simulink model "statsdem"  (Simulink 4.00)
settings: Solver=FixedStepDiscrete  StartTime=0.0  StopTime=inf  RelTol=1e-3  AbsTol=1e-6
libraries: dspbuff3 x4, dspstat3 x3, dspsrcs3 x2
settings Model: Creator=don  LastModifiedBy=schim  SaveTime=off  SaveOutput=off  LimitDataPoints=off  IntegerOverflowMsg=none  RTWOptions=-aRollThreshold=2  ExtModeTrigMode=oneshot  ExtModeArmWhenConnect=off  BlockReductionOpt=off

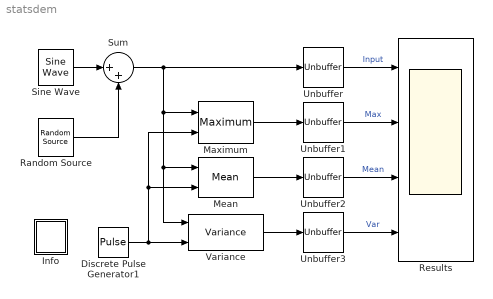
== system statsdem ==
  Discrete Pulse Generator1 : DiscretePulseGenerator  Amplitude=1  Period=100  PulseWidth=1  PhaseDelay=0  SampleTime=1
  Info : Subsystem
      settings: RTWFcnNameOpts=Auto  RTWFileNameOpts=Auto
      mask Display: disp('?')
  Maximum : dspstat3/Maximum  fcn=Running  reset=Non-zero sample
  Mean : dspstat3/Mean  run=on  reset_popup=Non-zero sample
  Random Source : dspsrcs3/Random Source  SrcType=Gaussian  Min=0  Max=1  Mean=0  Var=0.1  Seed=1  Inherit=off  SampMode=Discrete  SampTime=1/32  SampFrame=32  OutComplex=Real
  Results : Scope  NumInputPorts=4
      settings: TimeRange=100  YMin=-1.5~-0.25~-0.1~0  YMax=1.5~1.75~0.8~0.9  SaveToWorkspace=off  SaveName=ScopeData  DataFormat=Structure  LimitDataPoints=on  MaxDataPoints=1000
  Sine Wave : dspsrcs3/Sine Wave  Amplitude=1  Frequency=0.05  Phase=0  SampleMode=Discrete  OutComplex=Real  CompMethod=Trigonometric Fcn  SampleTime=1/32  SamplesPerFrame=32  ResetState=Restart at time zero
  Sum : Sum  Inputs=|++  SaturateOnIntegerOverflow=on
  Unbuffer{,1..3} (4 alike) : dspbuff3/Unbuffer  ic=0
  Variance : dspstat3/Variance  run=on  reset_popup=Non-zero sample
  wires:
  Discrete Pulse Generator1/1 -> Maximum/2, Mean/2, Variance/2
  Sum/1 -> Maximum/1, Mean/1, Variance/1, Unbuffer/1
  Random Source/1 -> Sum/2
  Sine Wave/1 -> Sum/1
  Maximum/1 -> Unbuffer1/1
  Mean/1 -> Unbuffer2/1
  Variance/1 -> Unbuffer3/1
  Unbuffer/1 -> Results/1  "Input"
  Unbuffer1/1 -> Results/2  "Max"
  Unbuffer2/1 -> Results/3  "Mean"
  Unbuffer3/1 -> Results/4  "Var"

== system statsdem/Info ==
  note: This demonstration model illustrates the behavior of
      | several running-statistics blocks which are
      | periodically reset after every 100 input samples.
      |
      | The model uses a noisy sine wave as the input to
      | each statistical function.
